simulink model "WhirlyBird_PID"  (R2016b)
settings: Solver=ode45  StartTime=0.0  StopTime=500  RelTol=1e-3  EnableMultiTasking=on
InitFcn:
  | param
undefined symbols (not defined in the file or in its folder): drawWhirly, P, whirly_ctrl, whirlyPWM
settings Model: Creator=beard  LastModifiedBy=Jacob
settings DataIOCC: LimitDataPoints=on  SaveFormat=Array  SignalLoggingSaveFormat=ModelDataLogs
settings OptimizationCC: ExpressionDepthLimit=2147483647  InitFltsAndDblsToZero=on  LifeSpan=inf
settings DebuggingCC: UnderspecifiedInitializationDetection=Classic  MergeDetectMultiDrivingBlocksExec=none  SolverPrmCheckMsg=warning  FcnCallInpInsideContextMsg=warning  StateNameClashWarn=warning  SFUnexpectedBacktrackingDiag=warning  SFNoUnconditionalDefaultTransitionDiag=warning  SFExecutionAtInitializationDiag=none
settings HardwareCC: ProdBitPerPointer=32  ProdBitPerSizeT=32  ProdBitPerPtrDiffT=32  ProdLargestAtomicFloat=None  ProdIntDivRoundTo=Undefined  ProdEndianess=Unspecified  ProdWordSize=32  ProdHWDeviceType=32-bit Generic
settings ModelReferenceCC: PropagateSignalLabelsOutOfModel=off
settings GRTTargetCC: TargetLangStandard=C89/C90 (ANSI)  GeneratePreprocessorConditionals=Disable all  CombineOutputUpdateFcns=off  GRTInterface=on
settings ConfigComp: CovMetricSettings=dw  CovHtmlReporting=on  CovSaveCumulativeToWorkspaceVar=on  CovSaveSingleToWorkspaceVar=on  CovExternalEMLEnable=off

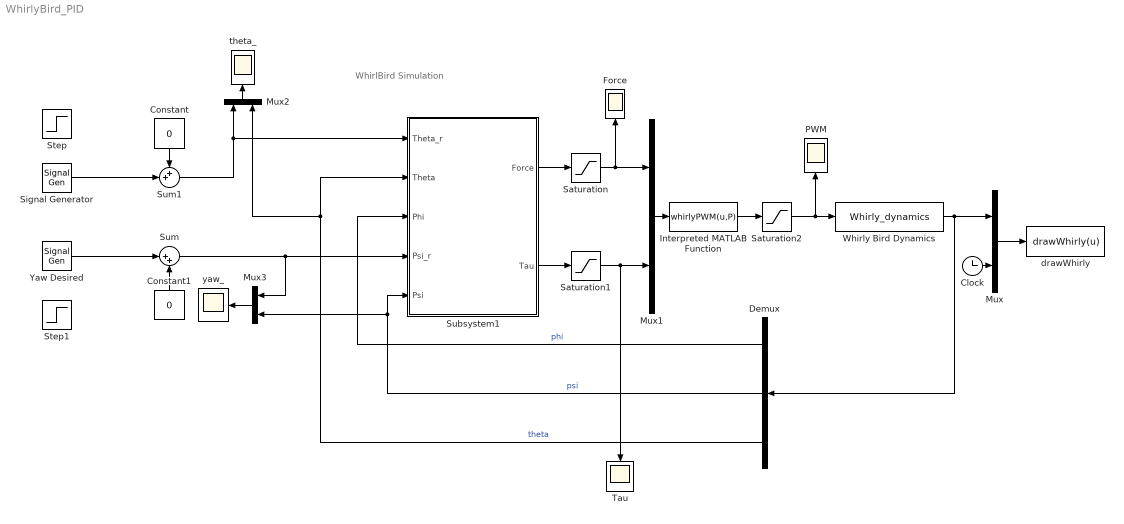
== system WhirlyBird_PID ==
  note: WhirlBird Simulation
  Clock : Clock
  Constant : Constant  Value=0
  Constant1 : Constant  Value=0
  Demux : Demux  Outputs=3
  Force : Scope
  Interpreted MATLAB Function : MATLABFcn  MATLABFcn=whirlyPWM(u,P)  OutputDimensions=2
  Mux{,1..3} (4 alike) : Mux  Inputs=2
  PWM : Scope
  Saturation : Saturate  UpperLimit=P.forcemax  LowerLimit=0
  Saturation1 : Saturate  UpperLimit=P.taumax  LowerLimit=-P.taumax
  Saturation2 : Saturate  UpperLimit=.6  LowerLimit=0
  Signal Generator : SignalGenerator  WaveForm=square  Amplitude=.2618*2  Frequency=.02
  Step : Step  Time=15  After=0.3  SampleTime=0
  Step1 : Step  Time=25  After=.5  SampleTime=0
  Subsystem1 : Subsystem
  Sum : Sum  Inputs=|++
  Sum1 : Sum  Inputs=++|
  Tau : Scope
  Whirly Bird Dynamics : S-Function  FunctionName=Whirly_dynamics  Parameters=P  SFunctionDeploymentMode=off  EnableBusSupport=off
  Yaw Desired : SignalGenerator  WaveForm=square  Amplitude=.2618*2  Frequency=.02
  drawWhirly : MATLABFcn  MATLABFcn=drawWhirly(u)  OutputDimensions=0  SampleTime=0.1
  theta_ : Scope
  yaw_ : Scope
  wires:
  Whirly Bird Dynamics/1 -> Mux/1, Demux/1
  Clock/1 -> Mux/2
  Mux/1 -> drawWhirly/1
  Mux2/1 -> theta_/1
  Mux1/1 -> Interpreted MATLAB Function/1
  Demux/3 -> Mux2/2, Subsystem1/2(Theta)  "theta"
  Saturation/1 -> Mux1/1, Force/1
  Demux/2 -> Subsystem1/5(Psi), Mux3/2  "psi"
  Mux3/1 -> yaw_/1
  Saturation1/1 -> Mux1/2, Tau/1
  Demux/1 -> Subsystem1/3(Phi)  "phi"
  Subsystem1/1(Force) -> Saturation/1
  Subsystem1/2(Tau) -> Saturation1/1
  Constant/1 -> Sum1/1
  Constant1/1 -> Sum/2
  Sum/1 -> Mux3/1, Subsystem1/4(Psi_r)
  Sum1/1 -> Mux2/1, Subsystem1/1(Theta_r)
  Interpreted MATLAB Function/1 -> Saturation2/1
  Yaw Desired/1 -> Sum/1
  Signal Generator/1 -> Sum1/2
  Saturation2/1 -> Whirly Bird Dynamics/1, PWM/1

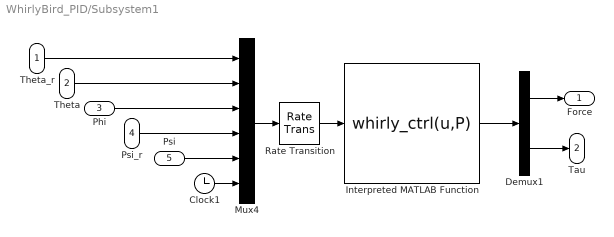
== system WhirlyBird_PID/Subsystem1 ==
  Theta_r : Inport
  Theta : Inport  Port=2
  Phi : Inport  Port=3
  Psi_r : Inport  Port=4
  Psi : Inport  Port=5
  Clock1 : Clock
  Demux1 : Demux  Outputs=2
  Interpreted MATLAB Function : MATLABFcn  MATLABFcn=whirly_ctrl(u,P)  OutputDimensions=2  Output1D=off
  Mux4 : Mux  Inputs=6
  Rate Transition : RateTransition  OutPortSampleTime=P.Ts
  Force : Outport
  Tau : Outport  Port=2
  wires:
  Theta_r/1 -> Mux4/1
  Psi/1 -> Mux4/5
  Psi_r/1 -> Mux4/4
  Theta/1 -> Mux4/2
  Clock1/1 -> Mux4/6
  Phi/1 -> Mux4/3
  Rate Transition/1 -> Interpreted MATLAB Function/1
  Mux4/1 -> Rate Transition/1
  Interpreted MATLAB Function/1 -> Demux1/1
  Demux1/1 -> Force/1
  Demux1/2 -> Tau/1
